simulink model "slip_ratio"  (R2015a)
settings: Solver=ode3  StartTime=0.0  StopTime=10.0  RelTol=1e-3
settings Model: Creator=BML  LastModifiedBy=BML
settings SolverCC: AutoInsertRateTranBlk=on

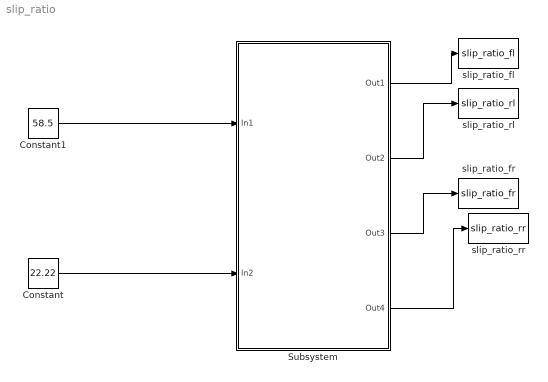
== system slip_ratio ==
  Constant : Constant  Value=22.22
  Constant1 : Constant  Value=58.5
  Subsystem : Subsystem
  slip_ratio_fl : ToWorkspace  VariableName=slip_ratio_fl  SaveFormat=Timeseries  SampleTime=-1
  slip_ratio_fr : ToWorkspace  VariableName=slip_ratio_fr  SaveFormat=Timeseries  SampleTime=-1
  slip_ratio_rl : ToWorkspace  VariableName=slip_ratio_rl  SaveFormat=Timeseries  SampleTime=-1
  slip_ratio_rr : ToWorkspace  VariableName=slip_ratio_rr  SaveFormat=Timeseries  SampleTime=-1
  wires:
  Constant1/1 -> Subsystem/1(In1)
  Constant/1 -> Subsystem/2(In2)
  Subsystem/1(Out1) -> slip_ratio_fl/1
  Subsystem/2(Out2) -> slip_ratio_rl/1
  Subsystem/3(Out3) -> slip_ratio_fr/1
  Subsystem/4(Out4) -> slip_ratio_rr/1

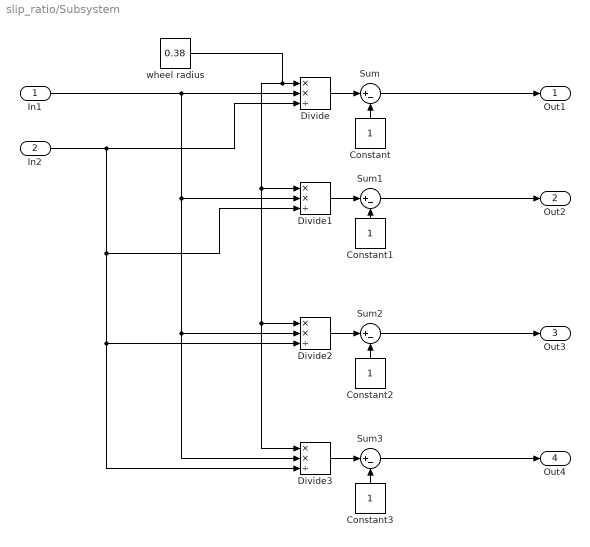
== system slip_ratio/Subsystem ==
  In1 : Inport
  In2 : Inport  Port=2
  Constant{,1..3} (4 alike) : Constant
  Divide{,1..3} (4 alike) : Product  Inputs=**/
  Sum{,1..3} (4 alike) : Sum  Inputs=|+-
  wheel radius : Constant  Value=0.38
  Out1 : Outport
  Out2 : Outport  Port=2
  Out3 : Outport  Port=3
  Out4 : Outport  Port=4
  wires:
  Constant/1 -> Sum/2
  Sum/1 -> Out1/1
  Divide1/1 -> Sum1/1
  Constant1/1 -> Sum1/2
  Divide/1 -> Sum/1
  Constant3/1 -> Sum3/2
  In1/1 -> Divide/2, Divide3/2, Divide2/2, Divide1/2
  In2/1 -> Divide3/3, Divide2/3, Divide1/3, Divide/3
  Sum1/1 -> Out2/1
  Divide2/1 -> Sum2/1
  Sum2/1 -> Out3/1
  Divide3/1 -> Sum3/1
  Sum3/1 -> Out4/1
  Constant2/1 -> Sum2/2
  wheel radius/1 -> Divide3/1, Divide2/1, Divide1/1, Divide/1
